simulink model "TP09_Ej08"  (R2020b)
settings: Solver=FixedStepAuto  StartTime=0.0  StopTime=2.5  FixedStep=1e-3  RelTol=1e-3
settings Model: Creator=Juan  LastModifiedBy=Juan

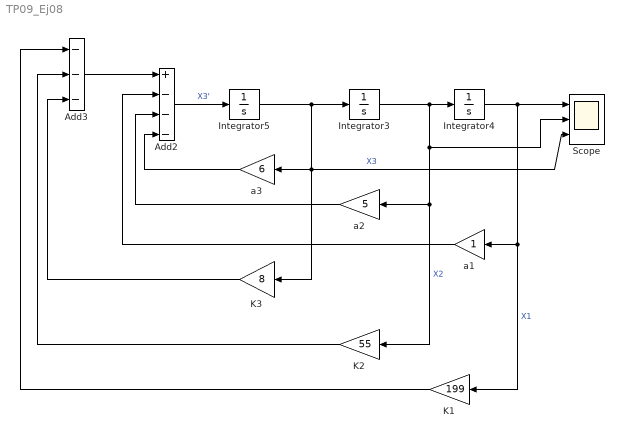
== system TP09_Ej08 ==
  Add2 : Sum  Inputs=+---
  Add3 : Sum  Inputs=---
  Integrator3 : Integrator
  Integrator4 : Integrator  InitialCondition=1
  Integrator5 : Integrator
  K1 : Gain  Gain=199
  K2 : Gain  Gain=55
  K3 : Gain  Gain=8
  Scope : Scope  NumInputPorts=3
  a1 : Gain
  a2 : Gain  Gain=5
  a3 : Gain  Gain=6
  wires:
  a1/1 -> Add2/2
  K3/1 -> Add3/3
  Add3/1 -> Add2/1
  Integrator4/1 -> Scope/1, K1/1, a1/1  "X1"
  K2/1 -> Add3/2
  Integrator3/1 -> Scope/2, K2/1, a2/1, Integrator4/1  "X2"
  a3/1 -> Add2/4
  a2/1 -> Add2/3
  Add2/1 -> Integrator5/1  "X3'"
  Integrator5/1 -> Integrator3/1, Scope/3, K3/1, a3/1  "X3"
  K1/1 -> Add3/1
